simulink library "TYPEC_MASTER"  (Simulink 8.6)
settings: Solver=ode45  StartTime=0.0  StopTime=10.0  RelTol=1e-3
libraries: STATE_BIO_MASTER x2, cdsEpicsBinIn x2, cdsFilt x2, cdsMuxMatrix x2, cdsEpicsStringIn x1, cdsDacKill x1, cdsEpicsOut x1, VIS_LIB x1, ISC_common x1, SIXOSEM_F_STAGE_MASTER x1, FOUROSEM_OPLEV_DAMP_MASTER x1, cdsEpicsMomentary x1
settings Model: Creator=keiko  LastModifiedBy=controls

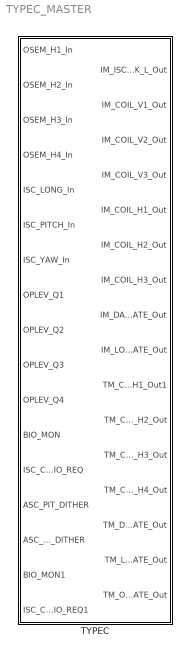
== system TYPEC_MASTER ==
  TYPEC : Subsystem  Description=TYPEC MASTER
      settings: AttributesFormatString=%<Description>

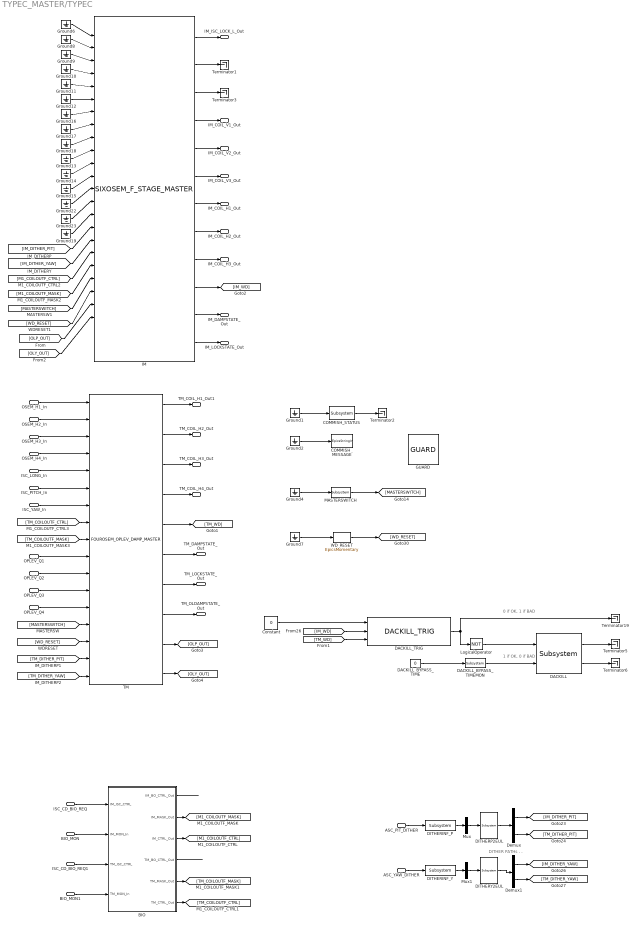
== system TYPEC_MASTER/TYPEC ==
  note: DITHER PATHs
      |
      |
      |
      |
      |
      |
      |
      |
      |
      |
      |
      |
      |
      |
      | .                                                                                                      .
  note: 1 if OK, 0 if BAD
  note: 0 if OK, 1 if BAD
  OSEM_H1_In : Inport
  OSEM_H2_In : Inport  Port=2
  OSEM_H3_In : Inport  Port=3
  OSEM_H4_In : Inport  Port=4
  ISC_LONG_In : Inport  Port=5
  ISC_PITCH_In : Inport  Port=6
  ISC_YAW_In : Inport  Port=7
  OPLEV_Q1 : Inport  Port=8
  OPLEV_Q2 : Inport  Port=9
  OPLEV_Q3 : Inport  Port=10
  OPLEV_Q4 : Inport  Port=11
  BIO_MON : Inport  Port=12
  ISC_CD_BIO_REQ : Inport  Port=13
  ASC_PIT_DITHER : Inport  Port=14
  ASC_YAW_DITHER : Inport  Port=15
  BIO_MON1 : Inport  Port=16
  ISC_CD_BIO_REQ1 : Inport  Port=17
  BIO : Subsystem
  COMMISH_MESSAGE : cdsEpicsStringIn/EpicsStringIn  Tag=cdsEpicsStringIn  Description=cdsEpicsStringIn
      settings: AttributesFormatString=%<Tag>
  COMMISH_STATUS : cdsEpicsBinIn/Subsystem  Tag=cdsEpicsBinIn  Description=|
      | Purpose:                                                                            
      | Create an EPICS binary (0 or 1) input channel to the FE realtime controls.          
      |                                                                                     
      | Operation:                                                                          
      | Outputs value from an EPICS ai record. Value is binary input (bi Epics record type).
      |                                                                                     
      | Usage:                                                                              
      | Name the part with the desired EPICS channel name.
      settings: AttributesFormatString=%<Tag>
  Constant : Constant  Value=0
  DACKILL : cdsDacKill/Subsystem  Description=cdsDacKill
      settings: AttributesFormatString=%<Description>
  DACKILL_BYPASS_TIME : Constant  Value=0
  DACKILL_BYPASS_TIMEMON : cdsEpicsOut/Subsystem  Tag=cdsEpicsOutput  Description=|
      | Purpose:                                          
      | Output a FE signal to an EPICS channel.           
      |                                                   
      | Operation:                                        
      | Takes input value and passes it to EPICS record.  
      |                                                   
      | Usage:                                            
      | Name the part with the desired EPICS rrecord name.
      settings: AttributesFormatString=%<Tag>
  DACKILL_TRIG : VIS_LIB/DACKILL_TRIG
  DITHERINF_P : cdsFilt/Subsystem  Tag=cdsFilt  Description=|
      | Purpose:                                                                                                                                                                                                                                  
      | Standard CDS IIR filter module.                                                                                                                                                                                                           
      |                                                                                                                                                                                                                                           
      | Operation:                                                                                                                                                                                                                                
      | Consists of 10 second order section IIR filters, plus a ramped gain stage. In FE code, also provides pre-defined test points and excitation channel inputs. The filter coefficients are defined in the LIGO system using the 'foton' tool.
      |                                                                                                                                                                                                                                           
      | Usage:                                                                                                                                                                                                                                    
      | Name the part with the desired filter module name.
      settings: AttributesFormatString=%<Tag>
  DITHERINF_Y : cdsFilt/Subsystem  Tag=cdsFilt  Description=|
      | Purpose:                                                                                                                                                                                                                                  
      | Standard CDS IIR filter module.                                                                                                                                                                                                           
      |                                                                                                                                                                                                                                           
      | Operation:                                                                                                                                                                                                                                
      | Consists of 10 second order section IIR filters, plus a ramped gain stage. In FE code, also provides pre-defined test points and excitation channel inputs. The filter coefficients are defined in the LIGO system using the 'foton' tool.
      |                                                                                                                                                                                                                                           
      | Usage:                                                                                                                                                                                                                                    
      | Name the part with the desired filter module name.
      settings: AttributesFormatString=%<Tag>
  DITHERP2EUL : cdsMuxMatrix/Subsystem  Tag=cdsMuxMatrix  Description=Any size matrix. Inputs and outputs must be connected using Mux and Demux parts.
      settings: AttributesFormatString=%<Tag>
  DITHERY2EUL : cdsMuxMatrix/Subsystem  Tag=cdsMuxMatrix  Description=Any size matrix. Inputs and outputs must be connected using Mux and Demux parts.
      settings: AttributesFormatString=%<Tag>
  Demux : Demux  Outputs=2
  Demux1 : Demux  Outputs=2
  GUARD : ISC_common/GUARD
  Ground{1..2,4,6..19,22..23} (19 alike) : Ground
  IM : SIXOSEM_F_STAGE_MASTER/SIXOSEM_F_STAGE_MASTER  Description=SIXOSEMSTAGE_FACE_MASTER
  LogicalOperator : Logic  Operator=NOT  AllPortsSameDT=off  OutDataTypeStr=boolean
  MASTERSWITCH : cdsEpicsBinIn/Subsystem  Tag=cdsEpicsBinIn  Description=|
      | Purpose:                                                                            
      | Create an EPICS binary (0 or 1) input channel to the FE realtime controls.          
      |                                                                                     
      | Operation:                                                                          
      | Outputs value from an EPICS ai record. Value is binary input (bi Epics record type).
      |                                                                                     
      | Usage:                                                                              
      | Name the part with the desired EPICS channel name.
      settings: AttributesFormatString=%<Tag>
  Mux : Mux  Inputs=1
  Mux1 : Mux  Inputs=1
  TM : FOUROSEM_OPLEV_DAMP_MASTER/FOUROSEM_OPLEV_DAMP_MASTER
  Terminator{1..3,5..6,19} (6 alike) : Terminator
  WD_RESET : cdsEpicsMomentary/EpicsMomentary  Tag=cdsEpicsMomentary
      settings: AttributesFormatString=%<Tag>
  IM_ISC_LOCK_L_Out : Outport
  IM_COIL_V1_Out : Outport  Port=2
  IM_COIL_V2_Out : Outport  Port=3
  IM_COIL_V3_Out : Outport  Port=4
  IM_COIL_H1_Out : Outport  Port=5
  IM_COIL_H2_Out : Outport  Port=6
  IM_COIL_H3_Out : Outport  Port=7
  IM_DAMPSTATE_Out : Outport  Port=8
  IM_LOCKSTATE_Out : Outport  Port=9
  TM_COIL_H1_Out1 : Outport  Port=10
  TM_COIL_H2_Out : Outport  Port=11
  TM_COIL_H3_Out : Outport  Port=12
  TM_COIL_H4_Out : Outport  Port=13
  TM_DAMPSTATE_Out : Outport  Port=14
  TM_LOCKSTATE_Out : Outport  Port=15
  TM_OLDAMPSTATE_Out : Outport  Port=16
  wires:
  [IM_WD] -> DACKILL_TRIG/2
  [TM_COILOUTF_MASK] -> TM/9
  [TM_COILOUTF_CTRL] -> TM/8
  BIO/4(TM_BO_CTRL_Out) -> ?
  BIO/6(TM_CTRL_Out) -> [TM_COILOUTF_CTRL]
  BIO/5(TM_MASK_Out) -> [TM_COILOUTF_MASK]
  ISC_CD_BIO_REQ1/1 -> BIO/3(TM_ISC_CTRL)
  BIO_MON1/1 -> BIO/4(TM_MON_In)
  [WD_RESET] -> TM/15
  WD_RESET/1 -> [WD_RESET]
  Ground7/1 -> WD_RESET/1
  TM/6 -> TM_DAMPSTATE_Out/1
  TM/7 -> TM_LOCKSTATE_Out/1
  TM/8 -> TM_OLDAMPSTATE_Out/1
  [MASTERSWITCH] -> TM/14
  OPLEV_Q4/1 -> TM/13
  ISC_YAW_In/1 -> TM/7
  ISC_PITCH_In/1 -> TM/6
  OPLEV_Q3/1 -> TM/12
  OPLEV_Q2/1 -> TM/11
  OPLEV_Q1/1 -> TM/10
  Ground4/1 -> MASTERSWITCH/1
  MASTERSWITCH/1 -> [MASTERSWITCH]
  ISC_CD_BIO_REQ/1 -> BIO/1(IM_ISC_CTRL)
  BIO_MON/1 -> BIO/2(IM_MON_In)
  BIO/1(IM_BO_CTRL_Out) -> ?
  BIO/2(IM_MASK_Out) -> [M1_COILOUTF_MASK]
  BIO/3(IM_CTRL_Out) -> [M1_COILOUTF_CTRL]
  TM/5 -> [TM_WD]
  ISC_LONG_In/1 -> TM/5
  OSEM_H4_In/1 -> TM/4
  OSEM_H3_In/1 -> TM/3
  OSEM_H2_In/1 -> TM/2
  OSEM_H1_In/1 -> TM/1
  Ground2/1 -> COMMISH_MESSAGE/1
  COMMISH_STATUS/1 -> Terminator2/1
  Ground1/1 -> COMMISH_STATUS/1
  ASC_YAW_DITHER/1 -> DITHERINF_Y/1
  Mux/1 -> DITHERP2EUL/1
  DITHERP2EUL/1 -> Demux/1
  ASC_PIT_DITHER/1 -> DITHERINF_P/1
  Mux1/1 -> DITHERY2EUL/1
  DITHERY2EUL/1 -> Demux1/1
  Demux/1 -> [IM_DITHER_PIT]
  Demux/2 -> [TM_DITHER_PIT]
  Demux1/1 -> [IM_DITHER_YAW]
  Demux1/2 -> [TM_DITHER_YAW]
  DITHERINF_P/1 -> Mux/1
  DITHERINF_Y/1 -> Mux1/1
  [TM_DITHER_PIT] -> TM/16
  [TM_DITHER_YAW] -> TM/17
  Ground9/1 -> IM/3
  Ground11/1 -> IM/5
  Ground17/1 -> IM/8
  Ground6/1 -> IM/1
  Ground8/1 -> IM/2
  Ground22/1 -> IM/13
  Ground10/1 -> IM/4
  Ground12/1 -> IM/6
  Ground23/1 -> IM/14
  Ground14/1 -> IM/11
  Ground16/1 -> IM/7
  Ground15/1 -> IM/12
  Ground19/1 -> IM/15
  Ground13/1 -> IM/10
  Ground18/1 -> IM/9
  [MASTERSWITCH] -> IM/20
  IM/1 -> IM_ISC_LOCK_L_Out/1
  IM/10 -> [IM_WD]
  IM/4 -> IM_COIL_V1_Out/1
  IM/5 -> IM_COIL_V2_Out/1
  IM/11 -> IM_DAMPSTATE_Out/1
  IM/2 -> Terminator1/1
  IM/3 -> Terminator3/1
  IM/6 -> IM_COIL_V3_Out/1
  IM/7 -> IM_COIL_H1_Out/1
  IM/9 -> IM_COIL_H3_Out/1
  IM/8 -> IM_COIL_H2_Out/1
  IM/12 -> IM_LOCKSTATE_Out/1
  DACKILL/2 -> Terminator6/1
  DACKILL/1 -> Terminator5/1
  DACKILL_BYPASS_TIME/1 -> DACKILL_BYPASS_TIMEMON/1
  DACKILL_BYPASS_TIMEMON/1 -> DACKILL/2
  LogicalOperator/1 -> DACKILL/1
  DACKILL_TRIG/1 -> Terminator19/1, LogicalOperator/1
  Constant/1 -> DACKILL_TRIG/1
  [TM_WD] -> DACKILL_TRIG/3
  TM/3 -> TM_COIL_H3_Out/1
  TM/4 -> TM_COIL_H4_Out/1
  TM/1 -> TM_COIL_H1_Out1/1
  TM/2 -> TM_COIL_H2_Out/1
  [IM_DITHER_PIT] -> IM/16
  [IM_DITHER_YAW] -> IM/17
  [M1_COILOUTF_CTRL] -> IM/18
  [M1_COILOUTF_MASK] -> IM/19
  [WD_RESET] -> IM/21
  [OLP_OUT] -> IM/22
  [OLY_OUT] -> IM/23
  TM/9 -> [OLP_OUT]
  TM/10 -> [OLY_OUT]

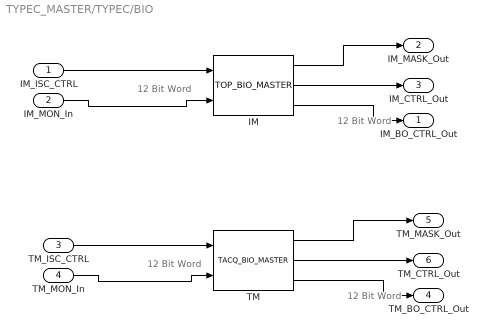
== system TYPEC_MASTER/TYPEC/BIO ==
  note: 12 Bit Word
  note: 12 Bit Word
  note: 12 Bit Word
  note: 12 Bit Word
  IM_ISC_CTRL : Inport
  IM_MON_In : Inport  Port=2
  TM_ISC_CTRL : Inport  Port=3
  TM_MON_In : Inport  Port=4
  IM : STATE_BIO_MASTER/TOP_BIO_MASTER
  TM : STATE_BIO_MASTER/TACQ_BIO_MASTER
  IM_BO_CTRL_Out : Outport
  IM_MASK_Out : Outport  Port=2
  IM_CTRL_Out : Outport  Port=3
  TM_BO_CTRL_Out : Outport  Port=4
  TM_MASK_Out : Outport  Port=5
  TM_CTRL_Out : Outport  Port=6
  wires:
  TM_ISC_CTRL/1 -> TM/1
  TM_MON_In/1 -> TM/2
  TM/3 -> TM_BO_CTRL_Out/1
  TM/1 -> TM_MASK_Out/1
  TM/2 -> TM_CTRL_Out/1
  IM_ISC_CTRL/1 -> IM/1
  IM_MON_In/1 -> IM/2
  IM/3 -> IM_BO_CTRL_Out/1
  IM/1 -> IM_MASK_Out/1
  IM/2 -> IM_CTRL_Out/1
